simulink model "s0103_Delta_ref_subsystem"  (R2021a)
settings: Solver=ode45  StartTime=0.0  StopTime=50  RelTol=1e-3
values from neighbouring files (symbols this model uses):
  ay_max = 9.9    [d0101_test_paramV2_data.mat]    (also in interpolation_test.m; m0101_test_paramV2_code.m)
  ay_nonLinear = 3.5    [d0101_test_paramV2_data.mat]    (also in m0101_test_paramV2_code.m)
  K_u = 0.105    [d0101_test_paramV2_data.mat]    (also in m0101_test_paramV2_code.m)
libraries: simulink x1
settings Model: Creator=asus  LastModifiedBy=ashli

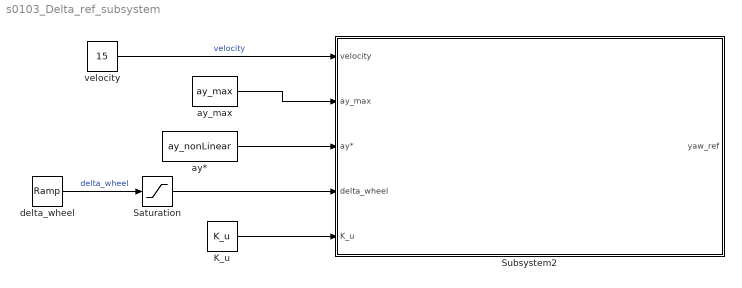
== system s0103_Delta_ref_subsystem ==
  K_u : Constant  Value=K_u
  Saturation : Saturate  UpperLimit=40.5
  Subsystem2 : Subsystem
  ay* : Constant  Value=ay_nonLinear
  ay_max : Constant  Value=ay_max
  delta_wheel : simulink/Sources/Ramp  slope=1  start=0  InitialOutput=0
  velocity : Constant  Value=15
  wires:
  velocity/1 -> Subsystem2/1(velocity)  "velocity"
  ay_max/1 -> Subsystem2/2(ay_max)
  ay*/1 -> Subsystem2/3(ay*)
  delta_wheel/1 -> Saturation/1  "delta_wheel"
  K_u/1 -> Subsystem2/5(K_u)
  Saturation/1 -> Subsystem2/4(delta_wheel)

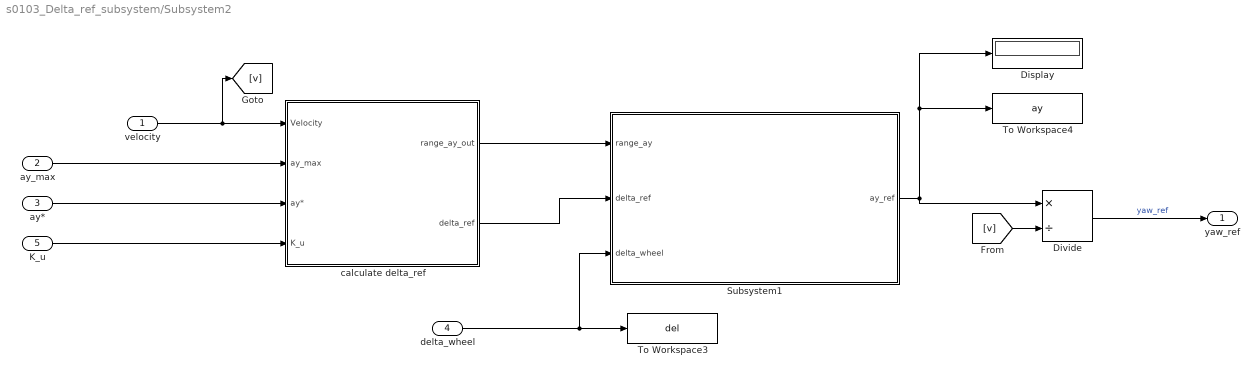
== system s0103_Delta_ref_subsystem/Subsystem2 ==
  velocity : Inport
  ay_max : Inport  Port=2
  ay* : Inport  Port=3
  delta_wheel : Inport  Port=4
  K_u : Inport  Port=5
  Display : Display
  Divide : Product  Inputs=*/
  Subsystem1 : Subsystem
  To Workspace3 : ToWorkspace  VariableName=del  SampleTime=-1
      settings: Save2DSignal=2-D array (concatenate along first dimension)
  To Workspace4 : ToWorkspace  VariableName=ay  SampleTime=-1
      settings: Save2DSignal=2-D array (concatenate along first dimension)
  calculate delta_ref : Subsystem
  yaw_ref : Outport
  wires:
  ay*/1 -> calculate delta_ref/3(ay*)
  Subsystem1/1(ay_ref) -> Display/1, To Workspace4/1, Divide/1
  delta_wheel/1 -> Subsystem1/3(delta_wheel), To Workspace3/1
  [v] -> Divide/2
  calculate delta_ref/1(range_ay_out) -> Subsystem1/1(range_ay)
  calculate delta_ref/2(delta_ref) -> Subsystem1/2(delta_ref)
  velocity/1 -> calculate delta_ref/1(Velocity), [v]
  ay_max/1 -> calculate delta_ref/2(ay_max)
  Divide/1 -> yaw_ref/1  "yaw_ref"
  K_u/1 -> calculate delta_ref/4(K_u)

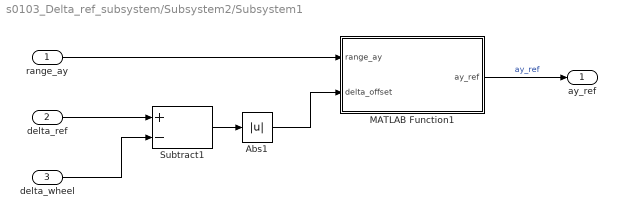
== system s0103_Delta_ref_subsystem/Subsystem2/Subsystem1 ==
  range_ay : Inport
  delta_ref : Inport  Port=2
  delta_wheel : Inport  Port=3
  Abs1 : Abs
  MATLAB Function1 : MATLAB Function  TreatAsAtomicUnit=on
  Subtract1 : Sum  Inputs=+-
  ay_ref : Outport
  wires:
  delta_wheel/1 -> Subtract1/2
  Subtract1/1 -> Abs1/1
  MATLAB Function1/1(ay_ref) -> ay_ref/1  "ay_ref"
  Abs1/1 -> MATLAB Function1/2(delta_offset)
  range_ay/1 -> MATLAB Function1/1(range_ay)
  delta_ref/1 -> Subtract1/1

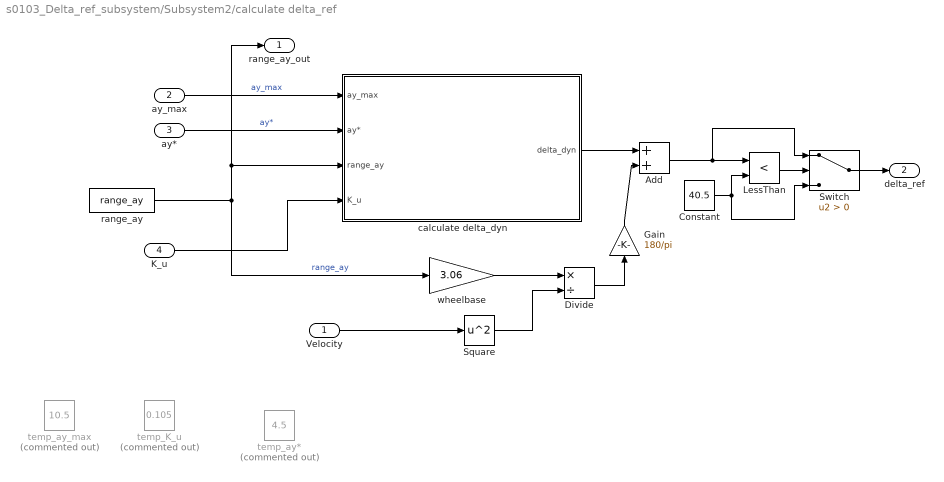
== system s0103_Delta_ref_subsystem/Subsystem2/calculate delta_ref ==
  Velocity : Inport
  ay_max : Inport  Port=2
  ay* : Inport  Port=3
  K_u : Inport  Port=4
  Add : Sum
  Constant : Constant  Value=40.5
  Divide : Product  Inputs=*/
  Gain : Gain  Gain=180/pi
  LessThan : RelationalOperator  Operator=<  OutDataTypeStr=boolean  RndMeth=Simplest
  Square : Math  Operator=square  SaturateOnIntegerOverflow=on
  Switch : Switch  Criteria=u2 > Threshold
  calculate delta_dyn : Subsystem
  range_ay : FromWorkspace  VariableName=range_ay  OutDataTypeStr=double
  temp_K_u : Constant  Commented=on  Value=0.105
  temp_ay* : Constant  Commented=on  Value=4.5
  temp_ay_max : Constant  Commented=on  Value=10.5
  wheelbase : Gain  Gain=3.06
  range_ay_out : Outport
  delta_ref : Outport  Port=2
  wires:
  range_ay/1 -> range_ay_out/1, calculate delta_dyn/3(range_ay), wheelbase/1  "range_ay"
  calculate delta_dyn/1(delta_dyn) -> Add/1
  wheelbase/1 -> Divide/1
  Velocity/1 -> Square/1
  Square/1 -> Divide/2
  Add/1 -> Switch/1, LessThan/1
  Divide/1 -> Gain/1
  Gain/1 -> Add/2
  Constant/1 -> Switch/3, LessThan/2
  LessThan/1 -> Switch/2
  Switch/1 -> delta_ref/1
  ay*/1 -> calculate delta_dyn/2(ay*)  "ay*"
  ay_max/1 -> calculate delta_dyn/1(ay_max)  "ay_max"
  K_u/1 -> calculate delta_dyn/4(K_u)

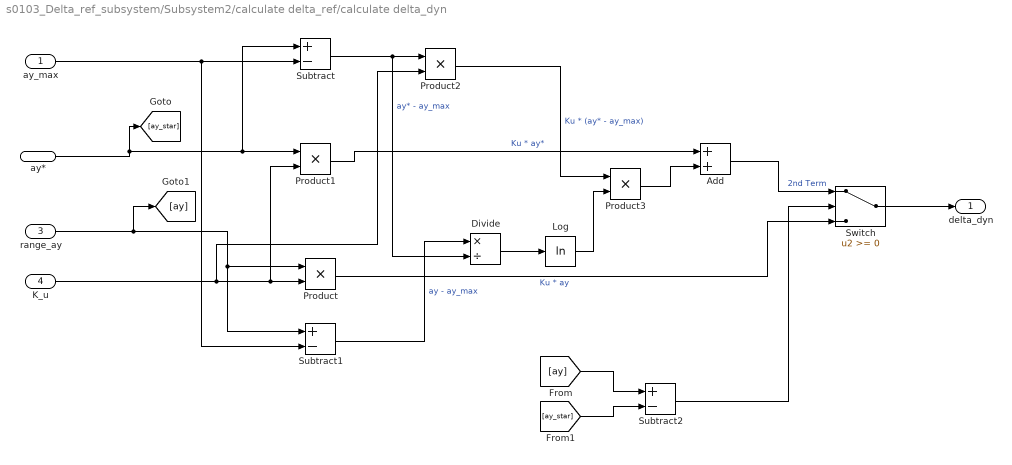
== system s0103_Delta_ref_subsystem/Subsystem2/calculate delta_ref/calculate delta_dyn ==
  ay_max : Inport
  ay* : Inport  Port=2
  range_ay : Inport  Port=3
  K_u : Inport  Port=4
  Add : Sum
  Divide : Product  Inputs=*/
  Log : Math  Operator=log  SaturateOnIntegerOverflow=on
  Product{,1..3} (4 alike) : Product
  Subtract : Sum  Inputs=+-
  Subtract1 : Sum  Inputs=+-
  Subtract2 : Sum  Inputs=+-
  Switch : Switch
  delta_dyn : Outport
  wires:
  Product2/1 -> Product3/1  "Ku * (ay* - ay_max)"
  Subtract/1 -> Divide/2, Product2/1  "ay* - ay_max"
  Log/1 -> Product3/2
  ay_max/1 -> Subtract/2, Subtract1/2
  Subtract1/1 -> Divide/1  "ay - ay_max"
  K_u/1 -> Product2/2, Product1/2, Product/2
  Add/1 -> Switch/1  "2nd Term"
  ay*/1 -> [ay_star], Subtract/1, Product1/1
  Divide/1 -> Log/1
  range_ay/1 -> [ay], Subtract1/1, Product/1
  Product3/1 -> Add/2
  Product1/1 -> Add/1  "Ku * ay*"
  [ay] -> Subtract2/1
  [ay_star] -> Subtract2/2
  Subtract2/1 -> Switch/2
  Product/1 -> Switch/3  "Ku * ay"
  Switch/1 -> delta_dyn/1

== matlab function s0103_Delta_ref_subsystem/Subsystem2/Subsystem1/MATLAB Function1 ==
  data: range_ay input; delta_offset input; ay_ref output
function ay_ref  = fcn(range_ay, delta_offset)

[val, pos] = min(delta_offset);
   
ay_ref = range_ay(pos);
